simulink model "main_system"  (R2015a)
settings: Solver=ode3  StartTime=0.0  StopTime=3  FixedStep=0.001  RelTol=1e-3
values from neighbouring files (symbols this model uses):
  simu_Gp = Gp2    [main.m]
undefined symbols (not defined in the file or in its folder): magnitude
libraries: simulink x1
settings Model: Creator=maen  LastModifiedBy=Xiaotian
settings DataIOCC: SignalLoggingSaveFormat=ModelDataLogs
settings OptimizationCC: ExpressionDepthLimit=2147483647
settings DebuggingCC: UnderspecifiedInitializationDetection=Classic  MergeDetectMultiDrivingBlocksExec=none  FcnCallInpInsideContextMsg=UseLocalSettings  StateNameClashWarn=warning
settings GRTTargetCC: CombineOutputUpdateFcns=off  GRTInterface=on

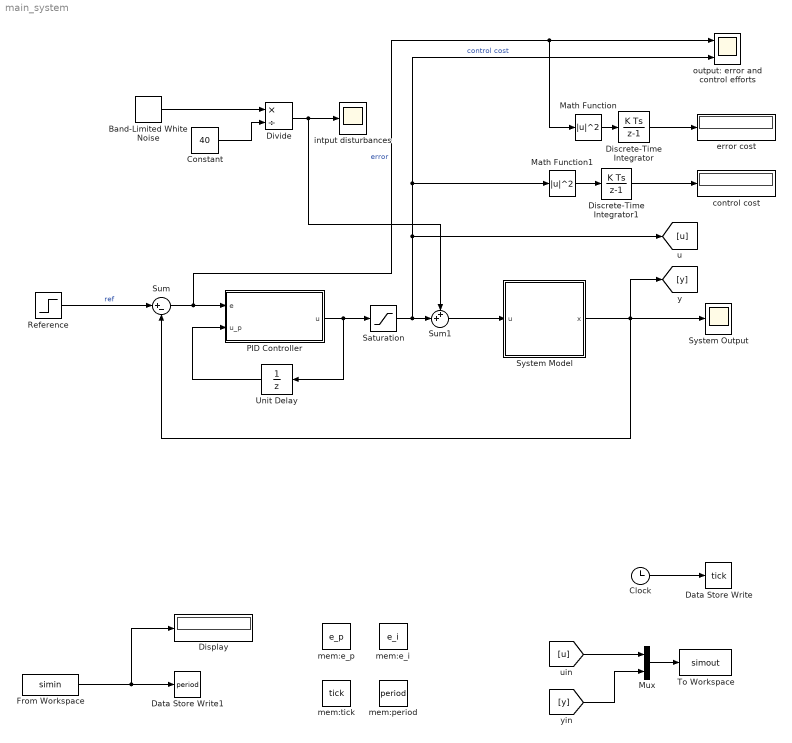
== system main_system ==
  Band-Limited White Noise : simulink/Sources/Band-Limited White Noise  Cov=simu_noise_power  Ts=0.001  seed=simu_noise_seed
  Clock : Clock
  Constant : Constant  Value=40
  Data Store Write : DataStoreWrite  DataStoreName=tick  SampleTime=0.001
  Data Store Write1 : DataStoreWrite  DataStoreName=period  SampleTime=0.001
  Discrete-Time Integrator : DiscreteIntegrator  InitialConditionSetting=State (most efficient)  SampleTime=0.001
  Discrete-Time Integrator1 : DiscreteIntegrator  InitialConditionSetting=State (most efficient)  SampleTime=0.001
  Display : Display
  Divide : Product  Inputs=*/
  From Workspace : FromWorkspace  VariableName=simin  SampleTime=0
  Math Function : Math  Operator=magnitude^2  SaturateOnIntegerOverflow=on
  Math Function1 : Math  Operator=magnitude^2  SaturateOnIntegerOverflow=on
  Mux : Mux  Inputs=2
  PID Controller : MATLAB Function  TreatAsAtomicUnit=on
  Reference : Step  Time=0  SampleTime=0
  Saturation : Saturate  UpperLimit=+12  LowerLimit=-12
  Sum : Sum  Inputs=|+-
  Sum1 : Sum  Inputs=++|
  System Model : Subsystem
  System Output : Scope
      settings: TickLabels=on  TimeRange=10  YMin=-0.4  YMax=1.4  MaxDataPoints=10000
  To Workspace : ToWorkspace  VariableName=simout  SaveFormat=Timeseries  SampleTime=-1
  Unit Delay : UnitDelay  SampleTime=-1
  control cost : Display
  error cost : Display
  intput disturbances : Scope
      settings: TickLabels=on  TimeRange=10  YMin=-40  YMax=40  SaveName=ScopeData2  MaxDataPoints=10000
  mem:e_i : DataStoreMemory  DataStoreName=e_i  OutDataTypeStr=double
  mem:e_p : DataStoreMemory  DataStoreName=e_p  OutDataTypeStr=double
  mem:period : DataStoreMemory  DataStoreName=period  OutDataTypeStr=double
  mem:tick : DataStoreMemory  DataStoreName=tick  OutDataTypeStr=double
  output: error and control efforts : Scope  NumInputPorts=2
      settings: TickLabels=on  TimeRange=3  YMin=0.95~-5  YMax=1.95~5  MaxDataPoints=10000
  wires:
  Clock/1 -> Data Store Write/1
  System Model/1(x) -> [y], Sum/2, System Output/1
  Sum/1 -> Math Function/1, output: error and control efforts/1, PID Controller/1(e)  "error"
  PID Controller/1(u) -> Saturation/1, Unit Delay/1
  Unit Delay/1 -> PID Controller/2(u_p)
  Sum1/1 -> System Model/1(u)
  Discrete-Time Integrator/1 -> error cost/1
  Discrete-Time Integrator1/1 -> control cost/1
  Math Function/1 -> Discrete-Time Integrator/1
  Math Function1/1 -> Discrete-Time Integrator1/1
  Mux/1 -> To Workspace/1
  From Workspace/1 -> Display/1, Data Store Write1/1
  Constant/1 -> Divide/2
  Band-Limited White Noise/1 -> Divide/1
  Divide/1 -> Sum1/1, intput disturbances/1
  Saturation/1 -> [u], output: error and control efforts/2, Math Function1/1, Sum1/2  "control cost"
  Reference/1 -> Sum/1  "ref"
  [u] -> Mux/1
  [y] -> Mux/2

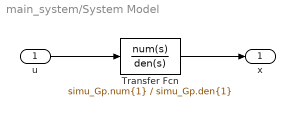
== system main_system/System Model ==
  u : Inport
  Transfer Fcn : TransferFcn  Numerator=simu_Gp.num{1}  Denominator=simu_Gp.den{1}
  x : Outport
  wires:
  u/1 -> Transfer Fcn/1
  Transfer Fcn/1 -> x/1

== matlab function main_system/PID Controller ==
  data: u output; e input; tick data_store_memory; u_p input; e_p data_store_memory; period data_store_memory; e_i data_store_memory
function u = fcn(e, u_p)

% parameters
simu_step = 0.001;      % simulation step

% global variables
global tick;
global e_p;             % previous error
global e_i;             % integrated error
global period;

% integrated error
e_i = e_i + e * period;

if ( mod(tick, period) <= simu_step )
    u = 10 * e + 5 * e_i + 0 * ((e - e_p) / period);
else
    u = u_p;
end

e_p = e;
